simulink model "three_phase_Fault_three_phase_loads_matlab_blockprevious"  (R2024a)
settings: Solver=VariableStepAuto  StartTime=0.0  StopTime=20  RelTol=1e-3
libraries: spsThreePhaseSeriesRLCLoadLib x3, spsThreePhaseVIMeasurementLib x3, spsThreePhaseBreakerLib x3, spsThreePhaseFaultLib x3, spsThreePhaseSourceLib x1, sps_lib x1
settings Model: SimulationMode=accelerator  Creator=Carnival  LastModifiedBy=Carnival

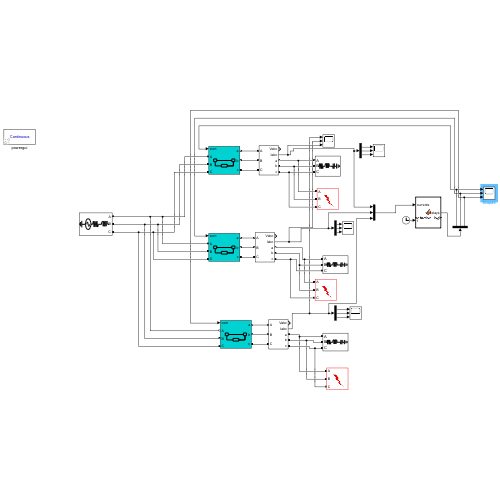
[thumbnail: Simulink's stored preview of the top-level diagram]
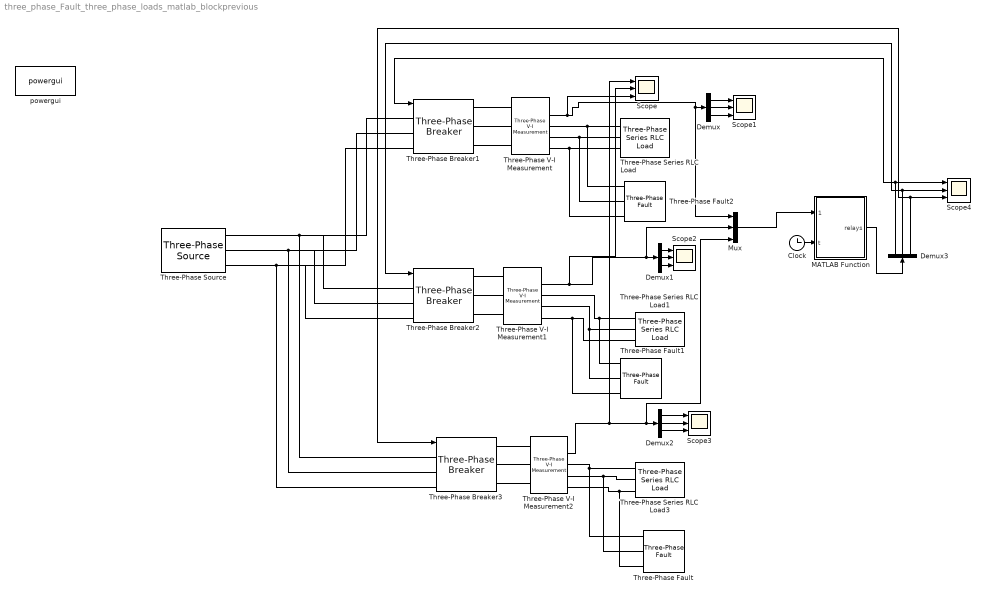
== system three_phase_Fault_three_phase_loads_matlab_blockprevious ==
  Clock : Clock
  Demux{,1..3} (4 alike) : Demux  Outputs=3
  MATLAB Function : MATLAB Function  TreatAsAtomicUnit=on
  Mux : Mux  Inputs=3
  Scope{,1..4} (5 alike) : Scope  NumInputPorts=3
  Three-Phase Series RLC Load : spsThreePhaseSeriesRLCLoadLib/Three-Phase Series RLC Load  LConnTagsString=A|B|C  Configuration=Y (grounded)  NominalVoltage=1000  Vabc=[1e3 1e3 1e3]  Vabcp=[1e3 1e3 1e3]  NominalFrequency=50  UnbalancedPower=off  ActivePower=10e3  InductivePower=100  CapacitivePower=100  Pabc=[10e3 9e3 11e3]  QLabc=[100 90 110]  QCabc=[100 90 110]  Pabcp=[10e3 9e3 11e3]  QLabcp=[100 90 110]  QCabcp=[100 90 110]  Measurements=None  LoadType=constant Z
  Three-Phase Series RLC Load1 : spsThreePhaseSeriesRLCLoadLib/Three-Phase Series RLC Load  LConnTagsString=A|B|C  Configuration=Y (grounded)  NominalVoltage=1000  Vabc=[1e3 1e3 1e3]  Vabcp=[1e3 1e3 1e3]  NominalFrequency=50  UnbalancedPower=off  ActivePower=10e3  InductivePower=100  CapacitivePower=100  Pabc=[10e3 9e3 11e3]  QLabc=[100 90 110]  QCabc=[100 90 110]  Pabcp=[10e3 9e3 11e3]  QLabcp=[100 90 110]  QCabcp=[100 90 110]  Measurements=None  LoadType=constant Z
  Three-Phase Series RLC Load3 : spsThreePhaseSeriesRLCLoadLib/Three-Phase Series RLC Load  LConnTagsString=A|B|C  Configuration=Y (grounded)  NominalVoltage=1000  Vabc=[1e3 1e3 1e3]  Vabcp=[1e3 1e3 1e3]  NominalFrequency=50  UnbalancedPower=off  ActivePower=10e3  InductivePower=100  CapacitivePower=100  Pabc=[10e3 9e3 11e3]  QLabc=[100 90 110]  QCabc=[100 90 110]  Pabcp=[10e3 9e3 11e3]  QLabcp=[100 90 110]  QCabcp=[100 90 110]  Measurements=None  LoadType=constant Z
  Three-Phase V-I Measurement : spsThreePhaseVIMeasurementLib/Three-Phase V-I Measurement  VoltageMeasurement=phase-to-ground  SetLabelV=off  LabelV=Vabc  Vpu=off  VpuLL=off  CurrentMeasurement=yes  SetLabelI=off  LabelI=Iabc  Ipu=off  Pbase=100e6  Vbase=500e3  OutputType=Complex  PhasorSimulation=off  PSBequivalent=0
  Three-Phase V-I Measurement1 : spsThreePhaseVIMeasurementLib/Three-Phase V-I Measurement  VoltageMeasurement=phase-to-ground  SetLabelV=off  LabelV=Vabc  Vpu=off  VpuLL=off  CurrentMeasurement=yes  SetLabelI=off  LabelI=Iabc  Ipu=off  Pbase=100e6  Vbase=500e3  OutputType=Complex  PhasorSimulation=off  PSBequivalent=0
  Three-Phase V-I Measurement2 : spsThreePhaseVIMeasurementLib/Three-Phase V-I Measurement  VoltageMeasurement=phase-to-ground  SetLabelV=off  LabelV=Vabc  Vpu=off  VpuLL=off  CurrentMeasurement=yes  SetLabelI=off  LabelI=Iabc  Ipu=off  Pbase=100e6  Vbase=500e3  OutputType=Complex  PhasorSimulation=off  PSBequivalent=0
  Three-Phase Breaker1 : spsThreePhaseBreakerLib/Three-Phase Breaker  InitialState=closed  SwitchA=on  SwitchB=on  SwitchC=on  SwitchTimes="[1/60  5/60]"  External=on  BreakerResistance=0.01  SnubberResistance=1e6  SnubberCapacitance=inf  Measurements=None
  Three-Phase Breaker2 : spsThreePhaseBreakerLib/Three-Phase Breaker  InitialState=closed  SwitchA=on  SwitchB=on  SwitchC=on  SwitchTimes="[1/60  5/60]"  External=on  BreakerResistance=0.01  SnubberResistance=1e6  SnubberCapacitance=inf  Measurements=None
  Three-Phase Breaker3 : spsThreePhaseBreakerLib/Three-Phase Breaker  InitialState=closed  SwitchA=on  SwitchB=on  SwitchC=on  SwitchTimes="[1/60  5/60]"  External=on  BreakerResistance=0.01  SnubberResistance=1e6  SnubberCapacitance=inf  Measurements=None
  Three-Phase Fault : spsThreePhaseFaultLib/Three-Phase Fault  InitialStates=0  FaultA=on  FaultB=on  FaultC=on  GroundFault=on  SwitchTimes="[10  11]"  External=off  SwitchStatus=NaN  FaultResistance=0.001  GroundResistance=0.01  SnubberResistance=1e6  SnubberCapacitance=inf  Measurements=None
  Three-Phase Fault1 : spsThreePhaseFaultLib/Three-Phase Fault  InitialStates=0  FaultA=on  FaultB=on  FaultC=on  GroundFault=on  SwitchTimes="[5  6]"  External=off  SwitchStatus=NaN  FaultResistance=0.001  GroundResistance=0.01  SnubberResistance=1e6  SnubberCapacitance=inf  Measurements=None
  Three-Phase Fault2 : spsThreePhaseFaultLib/Three-Phase Fault  InitialStates=0  FaultA=on  FaultB=on  FaultC=on  GroundFault=off  SwitchTimes="[1  2]"  External=off  SwitchStatus=NaN  FaultResistance=0.001  GroundResistance=0.01  SnubberResistance=1e6  SnubberCapacitance=inf  Measurements=None
  Three-Phase Source : spsThreePhaseSourceLib/Three-Phase Source  InternalConnection=Yg  VoltagePhases=off  Voltage=30  PhaseAngle=0  Voltage_phases=[25e3 25e3 25e3]/sqrt(3)  PhaseAngles_phases=[0 -120 +120]  Frequency=50  NonIdealSource=on  SpecifyImpedance=off  Resistance=0.8929  Inductance=16.58e-3  ShortCircuitLevel=100e6  BaseVoltage=25e3  XRratio=7  BusType=swing  Pref=10e3  Qref=0  Prefabc=[10e3, 10e3, 10e3]  Qrefabc=[0, 0, 0]  Qmin=-inf  Qmax=inf
  powergui : sps_lib/powergui  Priority=1  SimulationMode=Continuous  SampleTime=50e-6  frequency=60  Iterations=50  frequencyindice=50  Pbase=100e6  ErrMax=1e-4  UnitsV=kV  UnitsW=MW  buscounter=0  FunctionMessages=off  echomessages=off  EnableUseOfTLC=off  CurrentSourceSwitches=off  DisableSnubberDevices=off  DisableRonSwitches=off  DisableVfSwitches=off  DisplayEquations=off  AutomaticDiscreteSolvers=off  SolverType=Tustin/Backward Euler (TBE)  Interpol=off  ExternalGateDelay=off  methode=off  Ts=100  x0status=blocks  SPID=on  SwTol=0  HookPort=off  NonlinearTolerance=1e-4  nMaxIteration=100  ContinueOnMaxIteration=off  RestoreLinks=warning  ResistiveCurrentMeasurement=off  Frange=[0:2:500]  Ylog=off  Xlog=on  ShowGrid=off  save=off  variable=ZData  structure=0  ZoomFFT=off  StartTime=0.0  cycles=1  DisplayStyle=1  fundamental=60  FreqAxis=off  MaxFrequency=1000  frequencyindicesteady=1  RmsSteady=1  display=off
  wires:
  Three-Phase V-I Measurement/2 -> Scope/3, Mux/1, Demux/1
  Three-Phase V-I Measurement1/2 -> Scope/2, Mux/2, Demux1/1
  Three-Phase V-I Measurement2/2 -> Scope/1, Mux/3, Demux2/1
  Demux/1 -> Scope1/1
  Demux/2 -> Scope1/2
  Demux/3 -> Scope1/3
  Demux1/1 -> Scope2/1
  Demux1/2 -> Scope2/2
  Demux1/3 -> Scope2/3
  Demux2/1 -> Scope3/1
  Demux2/2 -> Scope3/2
  Demux2/3 -> Scope3/3
  Clock/1 -> MATLAB Function/2(t)
  Demux3/1 -> Three-Phase Breaker1/1, Scope4/1
  Demux3/2 -> Three-Phase Breaker2/1, Scope4/2
  Demux3/3 -> Three-Phase Breaker3/1, Scope4/3
  MATLAB Function/1(relays) -> Demux3/1
  Mux/1 -> MATLAB Function/1(currents)
  connections:
  Three-Phase Source/RConn1 -- Three-Phase Breaker2/LConn1 -- Three-Phase Breaker1/LConn1 -- Three-Phase Breaker3/LConn1
  Three-Phase Source/RConn2 -- Three-Phase Breaker2/LConn2 -- Three-Phase Breaker1/LConn2 -- Three-Phase Breaker3/LConn2
  Three-Phase Source/RConn3 -- Three-Phase Breaker2/LConn3 -- Three-Phase Breaker1/LConn3 -- Three-Phase Breaker3/LConn3
  Three-Phase Breaker1/RConn1 -- Three-Phase V-I Measurement/LConn1
  Three-Phase Breaker1/RConn2 -- Three-Phase V-I Measurement/LConn2
  Three-Phase Breaker1/RConn3 -- Three-Phase V-I Measurement/LConn3
  Three-Phase V-I Measurement/RConn1 -- Three-Phase Fault2/LConn1 -- Three-Phase Series RLC Load/LConn1
  Three-Phase Series RLC Load/LConn2 -- Three-Phase Fault2/LConn2 -- Three-Phase V-I Measurement/RConn2
  Three-Phase V-I Measurement/RConn3 -- Three-Phase Fault2/LConn3 -- Three-Phase Series RLC Load/LConn3
  Three-Phase V-I Measurement1/RConn3 -- Three-Phase Fault1/LConn3 -- Three-Phase Series RLC Load1/LConn3
  Three-Phase Breaker2/RConn3 -- Three-Phase V-I Measurement1/LConn3
  Three-Phase Series RLC Load1/LConn2 -- Three-Phase V-I Measurement1/RConn2 -- Three-Phase Fault1/LConn2
  Three-Phase Breaker2/RConn1 -- Three-Phase V-I Measurement1/LConn1
  Three-Phase Breaker2/RConn2 -- Three-Phase V-I Measurement1/LConn2
  Three-Phase V-I Measurement1/RConn1 -- Three-Phase Series RLC Load1/LConn1 -- Three-Phase Fault1/LConn1
  Three-Phase V-I Measurement2/RConn3 -- Three-Phase Fault/LConn3 -- Three-Phase Series RLC Load3/LConn3
  Three-Phase Breaker3/RConn3 -- Three-Phase V-I Measurement2/LConn3
  Three-Phase Series RLC Load3/LConn2 -- Three-Phase Fault/LConn2 -- Three-Phase V-I Measurement2/RConn2
  Three-Phase Breaker3/RConn1 -- Three-Phase V-I Measurement2/LConn1
  Three-Phase Breaker3/RConn2 -- Three-Phase V-I Measurement2/LConn2
  Three-Phase V-I Measurement2/RConn1 -- Three-Phase Fault/LConn1 -- Three-Phase Series RLC Load3/LConn1

== matlab function three_phase_Fault_three_phase_loads_matlab_blockprevious/MATLAB Function ==
  settings: updateMethod=DISCRETE
  data: currents input; relays output; t input
function relays = protection_logic(currents, t)

persistent fault_active reset_timer trip_start

if isempty(fault_active)
    fault_active = zeros(3,1);
    reset_timer  = zeros(3,1);
    trip_start   = -ones(3,1);
end

I_pickup = 0.3;
I_reset  = 1.5;
T_reset  = 0.05;
Ts       = 1e-4;

% --- IDMT constants ---
K   = 0.14;
n   = 0.02;
TMS = [0.1; 0.2; 0.3];

relays = ones(3,1);

for i = 1:3

    phases = currents((i-1)*3 + 1 : i*3);
    I_rms  = max(abs(phases));

    % =========================
    % --- IDMT Trip Logic ---
    % =========================
    if I_rms > I_pickup

        if trip_start(i) < 0
            trip_start(i) = t;   % start timing
        end

        ratio = I_rms / I_pickup;
        den   = (ratio^n - 1);

        if den > 0
            T_trip = TMS(i) * (K / den);
        else
            T_trip = inf;
        end

        if (t - trip_start(i)) >= T_trip
            fault_active(i) = 1;
            reset_timer(i)  = 0;
        end

    else
        trip_start(i) = -1;   % reset timing 
    end

    % =========================
    % --- Reset Logic ---
    % =========================
    if fault_active(i) == 1
        if I_rms < I_reset
            reset_timer(i) = reset_timer(i) + Ts;
            if reset_timer(i) >= T_reset
                fault_active(i) = 0;
                reset_timer(i)  = 0;
            end
        else
            reset_timer(i) = 0;
        end
    end

    % =========================
    % --- Output ---
    % =========================
    if fault_active(i) == 1
        relays(i) = 0;
    else
        relays(i) = 1;
    end

end

end
